simulink model "reprsentation_of_driver_drowsness_system_logic"  (R2021a)
settings: Solver=FixedStepAuto  StartTime=0.0  StopTime=inf  RelTol=1e-3
settings Model: EnablePacing=on  Creator=Beshary  LastModifiedBy=Beshary

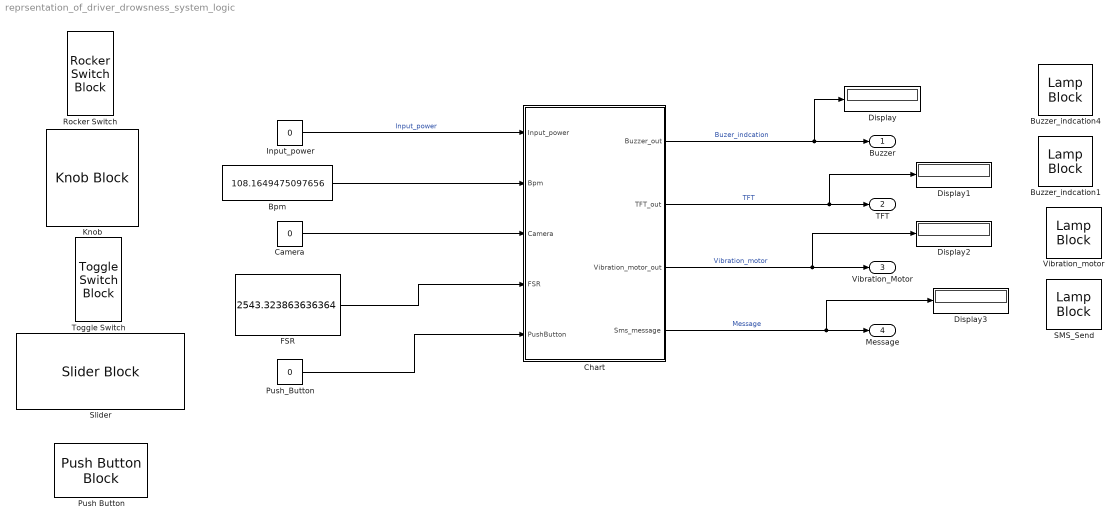
== system reprsentation_of_driver_drowsness_system_logic ==
  Bpm : Constant  Value=108.1649475097656
  Buzzer_indcation1 : LampBlock  Icon=LightingSwitch
  Buzzer_indcation4 : LampBlock  Icon=Hazards
  Camera : Constant  Value=0
  Chart : Stateflow chart  TreatAsAtomicUnit=on
  Display{,1..3} (4 alike) : Display
  FSR : Constant  Value=2543.323863636364
  Input_power : Constant  Value=0
  Knob : KnobBlock  ScaleMax=200
  Push Button : PushButtonBlock
  Push_Button : Constant  Value=0
  Rocker Switch : RockerSwitchBlock
      settings: Values={{'Off', 'On'}, [0 1]}
  SMS_Send : LampBlock  Icon=LightingSwitch
  Slider : SliderBlock  ScaleMin=500  ScaleMax=3000
  Toggle Switch : ToggleSwitchBlock
      settings: Values={{'Off', 'On'}, [0 1]}
  Vibration_motor : LampBlock  Icon=LightingSwitch
  Buzzer : Outport
  TFT : Outport  Port=2
  Vibration_Motor : Outport  Port=3
  Message : Outport  Port=4
  wires:
  Bpm/1 -> Chart/2(Bpm)
  Camera/1 -> Chart/3(Camera)
  Input_power/1 -> Chart/1(Input_power)  "Input_power"
  FSR/1 -> Chart/4(FSR)
  Chart/4(Sms_message) -> Display3/1, Message/1  "Message"
  Chart/3(Vibration_motor_out) -> Display2/1, Vibration_Motor/1  "Vibration_motor"
  Chart/2(TFT_out) -> Display1/1, TFT/1  "TFT"
  Chart/1(Buzzer_out) -> Display/1, Buzzer/1  "Buzer_indcation"
  Push_Button/1 -> Chart/5(PushButton)

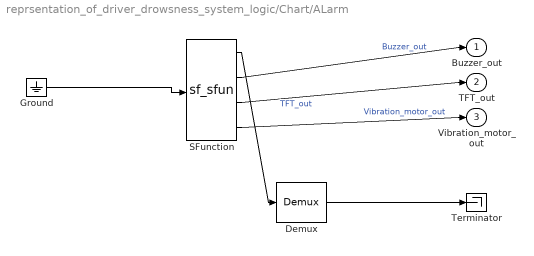
== system reprsentation_of_driver_drowsness_system_logic/Chart/ALarm ==
  " Demux " : Demux  Outputs=1
  " Ground " : Ground
  " SFunction " : S-Function  Tag=Stateflow S-Function 1  FunctionName=sf_sfun  PortCounts=[1 4]  SFunctionDeploymentMode=off  EnableBusSupport=off
  " Terminator " : Terminator
  Buzzer_out : Outport
  TFT_out : Outport  Port=2
  Vibration_motor_out : Outport  Port=3
  wires:
  " SFunction "/2 -> Buzzer_out/1  "Buzzer_out"
  " SFunction "/3 -> TFT_out/1  "TFT_out"
  " SFunction "/4 -> Vibration_motor_out/1  "Vibration_motor_out"
  " Ground "/1 -> " SFunction "/1
  " Demux "/1 -> " Terminator "/1
  " SFunction "/1 -> " Demux "/1

== stateflow chart reprsentation_of_driver_drowsness_system_logic/Chart/ALarm ==
  state Buzzer [parallel]
    en:
    Buzzer_out=1;
    settings: executionOrder=2
  state vibration_motor [parallel]
    en:
    Vibration_motor_out=1;
    settings: executionOrder=1
  state TFT [parallel]
    en:
    TFT_out=1;
    settings: executionOrder=3
  data: Buzzer_out output double; TFT_out output double; Vibration_motor_out output double

== stateflow chart reprsentation_of_driver_drowsness_system_logic/Chart ==
  state ALarm
  state Device_ON
    en:
  state Device_OFF
  state SMS
    en:
    Sms_message=1;
    ex:
    Sms_message=0;
  (default) -> Device_OFF
  ALarm -> Device_ON [order 1] : [PushButton==1]{Buzzer_out=0,Vibration_motor_out=0,TFT_out=0}
  Device_ON -> Device_OFF [order 1] : [Input_power==0]
  Device_ON -> ALarm [order 2] : [(FSR<2500)||(Camera==1)||(Bpm< 60||Bpm>140)]
  Device_OFF -> Device_ON : [Input_power==1]
  SMS -> Device_ON : [PushButton==1||Input_power==0]{Buzzer_out=0,Vibration_motor_out=0,TFT_out=0}
  ALarm -> SMS [order 2] : [((FSR<2500)||(Camera==1)||(Bpm< 60||Bpm>140))&&after(5,sec)]
  data: Input_power input; Bpm input; Camera input; FSR input; PushButton input; Buzzer_out output double; TFT_out output double; Vibration_motor_out output double; Sms_message output double
